simulink model "minmax_multi_test"  (Simulink 9.0)
settings: Solver=FixedStepAuto  StartTime=0.0  StopTime=10.0  FixedStep=0.1  RelTol=1e-3  EnableMultiTasking=on
settings Model: SuppressorTable=22 serialization::archive 11 0 6 0 0 0 0 0  Creator=arnaud  LastModifiedBy=hbourbou
settings DataIOCC: LimitDataPoints=on  SaveFormat=Structure  SignalLoggingSaveFormat=ModelDataLogs
settings OptimizationCC: ExpressionDepthLimit=2147483647
settings DebuggingCC: SolverPrmCheckMsg=warning  FcnCallInpInsideContextMsg=warning  StateNameClashWarn=warning  StrictBusMsg=Warning
settings GRTTargetCC: CombineOutputUpdateFcns=off  GRTInterface=on

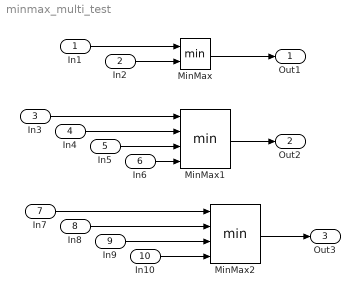
== system minmax_multi_test ==
  In1 : Inport  PortDimensions=1
  In2 : Inport  Port=2  PortDimensions=5
  In3 : Inport  Port=3  PortDimensions=1
  In4 : Inport  Port=4  PortDimensions=3
  In5 : Inport  Port=5  PortDimensions=3
  In6 : Inport  Port=6  PortDimensions=3
  In7 : Inport  Port=7  PortDimensions=1
  In8 : Inport  Port=8  PortDimensions=1
  In9 : Inport  Port=9  PortDimensions=[2 3]
  In10 : Inport  Port=10  PortDimensions=[2 3]
  MinMax : MinMax  Inputs=2
  MinMax1 : MinMax  Inputs=4
  MinMax2 : MinMax  Inputs=4
  Out1 : Outport
  Out2 : Outport  Port=2
  Out3 : Outport  Port=3
  wires:
  MinMax/1 -> Out1/1
  In1/1 -> MinMax/1
  In2/1 -> MinMax/2
  MinMax1/1 -> Out2/1
  In3/1 -> MinMax1/1
  In4/1 -> MinMax1/2
  In5/1 -> MinMax1/3
  In6/1 -> MinMax1/4
  MinMax2/1 -> Out3/1
  In7/1 -> MinMax2/1
  In8/1 -> MinMax2/2
  In9/1 -> MinMax2/3
  In10/1 -> MinMax2/4
